simulink model "konser"  (Simulink 8.3)
settings: Solver=ode3  StartTime=0.0  StopTime=simulation_time  FixedStep=dt  RelTol=1e-5
values from neighbouring files (symbols this model uses):
  k = 5    [programm.m]
  T = 0.1    [programm.m]
  w = w_1(j)    [programm.m]
settings Model: Creator=Павел  LastModifiedBy=Павел
settings DataIOCC: LimitDataPoints=off  SignalLoggingSaveFormat=Dataset
settings DebuggingCC: UnderspecifiedInitializationDetection=Simplified  StateNameClashWarn=none
settings GRTTargetCC: CombineOutputUpdateFcns=on  GRTInterface=off

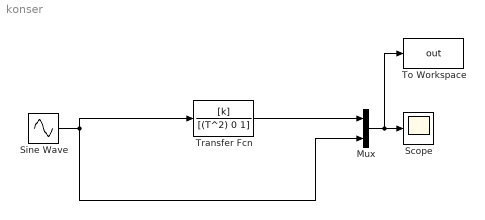
== system konser ==
  Mux : Mux  Inputs=2
  Scope : Scope
  Sine Wave : Sin  Frequency=w  SampleTime=0
  To Workspace : ToWorkspace  VariableName=out  SaveFormat=Structure With Time  SampleTime=-1
  Transfer Fcn : TransferFcn  Numerator=[k]  Denominator=[(T^2) 0 1]
  wires:
  Mux/1 -> To Workspace/1, Scope/1
  Sine Wave/1 -> Transfer Fcn/1, Mux/2
  Transfer Fcn/1 -> Mux/1
